simulink model "PSOCDerate"  (R2024b)
settings: configuration reference "STM32H7_Config" (kept outside this file)
settings Model: DataDictionary=Master_Dictionary.sldd  EnableAccessToBaseWorkspace=off  Creator=torni  LastModifiedBy=Will
settings ConfigSetRef: SourceName=STM32H7_Config

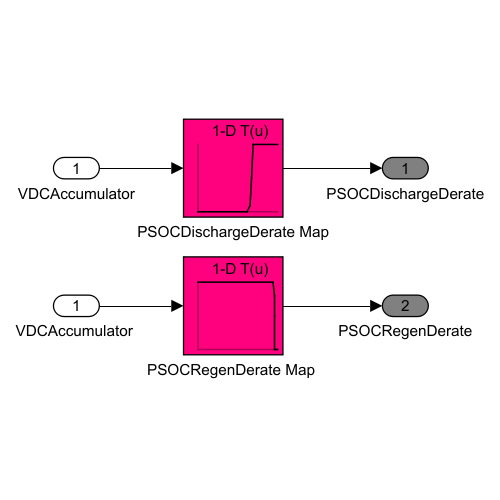
[thumbnail: Simulink's stored preview of the top-level diagram]
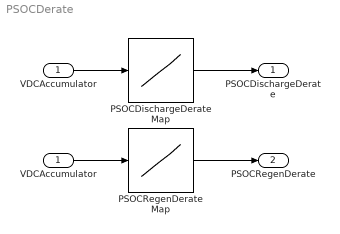
== system PSOCDerate ==
  VDCAccumulator : Inport  OutDataTypeStr=double
  PSOCDischargeDerate Map : Lookup_n-D  NumberOfTableDimensions=1  BreakpointsForDimension1=[0,377,390,403,416,600]  Table=[0,0,7.8,39,78,78]  InternalRulePriority=Speed  RndMeth=Simplest
  "PSOCRegenDerate Map " : Lookup_n-D  NumberOfTableDimensions=1  BreakpointsForDimension1=[0,569,574,576,578,600]  Table=[100,100,80,50,0,0]  InternalRulePriority=Speed  RndMeth=Simplest
  "VDCAccumulator " : InportShadow  OutDataTypeStr=double
  PSOCDischargeDerate : Outport  OutDataTypeStr=double  VectorParamsAs1DForOutWhenUnconnected=off
  PSOCRegenDerate : Outport  Port=2  OutDataTypeStr=double  VectorParamsAs1DForOutWhenUnconnected=off
  wires:
  VDCAccumulator/1 -> PSOCDischargeDerate Map/1
  PSOCDischargeDerate Map/1 -> PSOCDischargeDerate/1
  "PSOCRegenDerate Map "/1 -> PSOCRegenDerate/1
  "VDCAccumulator "/1 -> "PSOCRegenDerate Map "/1
